simulink model "Lab6_task"  (R2021a)
settings: Solver=VariableStepAuto  StartTime=0.0  StopTime=10.0  RelTol=1e-3
libraries: dspsrcs4 x3
settings Model: Creator=Syed Mujahid Abbas  LastModifiedBy=hp
settings SolverCC: AlgebraicLoopSolver=TrustRegion
settings DataIOCC: ReturnWorkspaceOutputs=off
settings DebuggingCC: SFMachineParentedDataDiag=warning  ArithmeticOperatorsInVariantConditions=warning
settings SFSimCC: SimUseLocalCustomCode=off  CustomCodeUndefinedFunction=UseInterfaceOnly
settings RTWCC: RTWUseLocalCustomCode=off

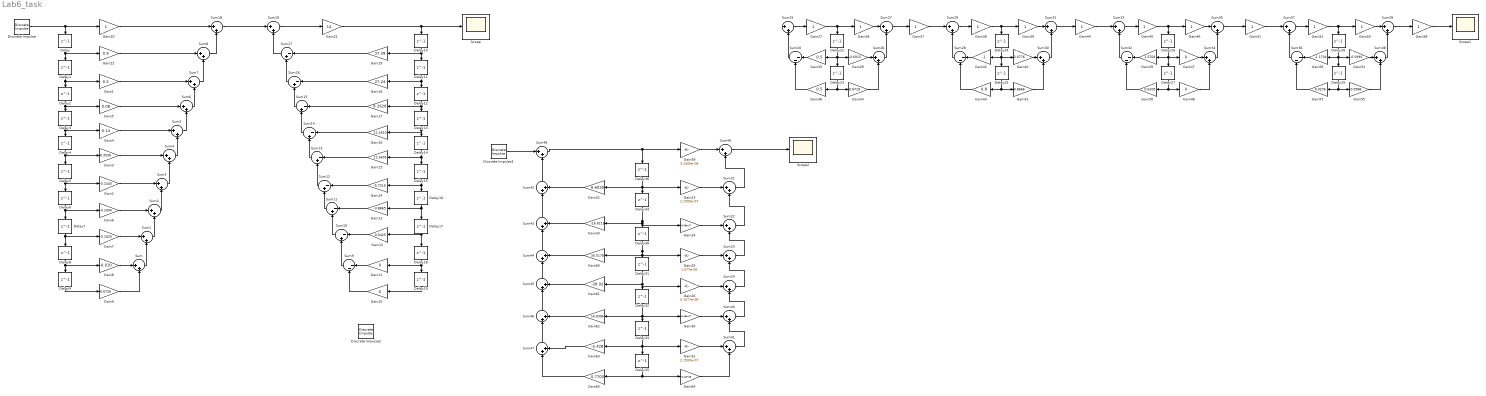
== system Lab6_task ==
  Delay{,1..19,22..36} (35 alike) : Delay  DelayLength=1  InitialCondition=0
  Discrete Impulse : dspsrcs4/Discrete  Impulse  Delay=0  SampleTime=1  FrameSample=1  OutputFrames=off  dataType=double  isSigned=on  wordLen=16  udDataType=sfix(16)  fracBitsMode=Best precision  numFracBits=15  OutDataTypeStr=double  LastOutDataTypeStr=double
  Discrete Impulse2 : dspsrcs4/Discrete  Impulse  Delay=0  SampleTime=1  FrameSample=1  OutputFrames=off  dataType=double  isSigned=on  wordLen=16  udDataType=sfix(16)  fracBitsMode=Best precision  numFracBits=15  OutDataTypeStr=double  LastOutDataTypeStr=double
  Discrete Impulse3 : dspsrcs4/Discrete  Impulse  Delay=0  SampleTime=1  FrameSample=1  OutputFrames=off  dataType=double  isSigned=on  wordLen=16  udDataType=sfix(16)  fracBitsMode=Best precision  numFracBits=15  OutDataTypeStr=double  LastOutDataTypeStr=double
  Gain1 : Gain  Gain=0.5
  Gain{10..11,47..48} (4 alike) : Gain  Gain=0
  Gain12 : Gain  Gain=0.5425
  Gain13 : Gain  Gain=-3.8865
  Gain14 : Gain  Gain=-5.7215
  Gain15 : Gain  Gain=11.6605
  Gain16 : Gain  Gain=12.4810
  Gain17 : Gain  Gain=6.2620
  Gain18 : Gain  Gain=27.24
  Gain19 : Gain  Gain=37.39
  Gain2 : Gain  Gain=-0.2440
  Gain{20,27..28,37..39,44..46,51..53,58} (13 alike) : Gain
  Gain21 : Gain  Gain=14
  Gain22 : Gain  Gain=0.9
  Gain23 : Gain  Gain=2.1500e-07
  Gain24 : Gain  Gain=6.46e-07
  Gain25 : Gain  Gain=1.077e-06
  Gain26 : Gain  Gain=0.1077e-06
  Gain29 : Gain  Gain=-0.6915
  Gain3 : Gain  Gain=0.3530
  Gain30 : Gain  Gain=6.46e-07
  Gain31 : Gain  Gain=2.1500e-07
  Gain32 : Gain  Gain=6.6030
  Gain33 : Gain  Gain=-18.8215
  Gain34 : Gain  Gain=0.6719
  Gain35 : Gain  Gain=0.5
  Gain36 : Gain  Gain=0.5
  Gain4 : Gain  Gain=0.14
  Gain40 : Gain  Gain=2.0776
  Gain41 : Gain  Gain=0.8666
  Gain42 : Gain  Gain=-1
  Gain43 : Gain  Gain=0.8
  Gain49 : Gain  Gain=1.5704
  Gain5 : Gain  Gain=0.08
  Gain50 : Gain  Gain=0.6105
  Gain54 : Gain  Gain=-0.5990
  Gain55 : Gain  Gain=0.0588
  Gain56 : Gain  Gain=-1.1704
  Gain57 : Gain  Gain=0.3276
  Gain59 : Gain  Gain=3.1000e-08
  Gain6 : Gain  Gain=-0.2890
  Gain60 : Gain  Gain=30.0178
  Gain61 : Gain  Gain=-28.92
  Gain62 : Gain  Gain=16.8386
  Gain63 : Gain  Gain=-5.428
  Gain64 : Gain  Gain=3.11e-08
  Gain65 : Gain  Gain=0.7703
  Gain7 : Gain  Gain=-0.1820
  Gain8 : Gain  Gain=-0.010
  Gain9 : Gain  Gain=0.0720
  Scope : Scope
  Scope1 : Scope
  Scope2 : Scope
  Sum{,1..8,18..19,21..27,29..31,33..35,37..49} (37 alike) : Sum  Inputs=|++
  Sum{10..17} (8 alike) : Sum  Inputs=|-+
  Sum{9,20,28,32,36} (5 alike) : Sum  Inputs=|--
  wires:
  Delay6/1 -> Delay7/1, Gain6/1
  Delay5/1 -> Gain2/1, Delay6/1
  Delay9/1 -> Gain9/1
  Delay8/1 -> Gain8/1, Delay9/1
  Delay7/1 -> Gain7/1, Delay8/1
  Sum/1 -> Sum1/2
  Gain6/1 -> Sum2/1
  Sum1/1 -> Sum2/2
  Delay4/1 -> Gain3/1, Delay5/1
  Delay3/1 -> Gain4/1, Delay4/1
  Delay2/1 -> Gain5/1, Delay3/1
  Delay1/1 -> Gain1/1, Delay2/1
  Delay/1 -> Gain22/1, Delay1/1
  Sum2/1 -> Sum3/2
  Gain2/1 -> Sum3/1
  Sum3/1 -> Sum4/2
  Sum4/1 -> Sum5/2
  Sum5/1 -> Sum6/2
  Sum6/1 -> Sum7/2
  Sum7/1 -> Sum8/2
  Delay18/1 -> Gain11/1, Delay19/1
  Delay19/1 -> Gain10/1
  Delay17/1 -> Gain12/1, Delay18/1
  Delay16/1 -> Gain13/1, Delay17/1
  Delay15/1 -> Gain14/1, Delay16/1
  Delay14/1 -> Gain15/1, Delay15/1
  Delay13/1 -> Gain16/1, Delay14/1
  Delay12/1 -> Gain17/1, Delay13/1
  Delay11/1 -> Gain18/1, Delay12/1
  Delay10/1 -> Gain19/1, Delay11/1
  Sum9/1 -> Sum10/2
  Sum10/1 -> Sum11/2
  Sum11/1 -> Sum12/2
  Sum12/1 -> Sum13/2
  Sum13/1 -> Sum14/2
  Sum14/1 -> Sum15/2
  Sum15/1 -> Sum16/2
  Sum16/1 -> Sum17/2
  Sum8/1 -> Sum18/2
  Sum17/1 -> Sum19/2
  Sum18/1 -> Sum19/1
  Discrete Impulse/1 -> Delay/1, Gain20/1
  Sum19/1 -> Gain21/1
  Gain3/1 -> Sum4/1
  Gain4/1 -> Sum5/1
  Gain5/1 -> Sum6/1
  Gain1/1 -> Sum7/1
  Gain22/1 -> Sum8/1
  Gain20/1 -> Sum18/1
  Gain7/1 -> Sum1/1
  Gain8/1 -> Sum/1
  Gain9/1 -> Sum/2
  Gain21/1 -> Delay10/1, Scope/1
  Gain10/1 -> Sum9/2
  Gain11/1 -> Sum9/1
  Gain12/1 -> Sum10/1
  Gain13/1 -> Sum11/1
  Gain14/1 -> Sum12/1
  Gain15/1 -> Sum13/1
  Gain16/1 -> Sum14/1
  Gain17/1 -> Sum15/1
  Gain18/1 -> Sum16/1
  Gain19/1 -> Sum17/1
  Sum26/1 -> Sum27/2
  Gain28/1 -> Sum27/1
  Gain34/1 -> Sum26/2
  Gain29/1 -> Sum26/1
  Sum25/1 -> Gain27/1
  Sum20/1 -> Sum25/2
  Gain35/1 -> Sum20/1
  Gain36/1 -> Sum20/2
  Delay23/1 -> Gain34/1, Gain36/1
  Delay22/1 -> Delay23/1, Gain29/1, Gain35/1
  Gain27/1 -> Gain28/1, Delay22/1
  Gain38/1 -> Delay24/1, Gain39/1
  Delay24/1 -> Gain42/1, Gain40/1, Delay25/1
  Delay25/1 -> Gain43/1, Gain41/1
  Gain43/1 -> Sum28/2
  Gain42/1 -> Sum28/1
  Gain37/1 -> Sum29/1
  Sum28/1 -> Sum29/2
  Sum29/1 -> Gain38/1
  Gain40/1 -> Sum30/1
  Gain41/1 -> Sum30/2
  Gain39/1 -> Sum31/1
  Sum30/1 -> Sum31/2
  Sum27/1 -> Gain37/1
  Sum34/1 -> Sum35/2
  Gain46/1 -> Sum35/1
  Gain48/1 -> Sum34/2
  Gain47/1 -> Sum34/1
  Sum33/1 -> Gain45/1
  Sum32/1 -> Sum33/2
  Gain44/1 -> Sum33/1
  Gain49/1 -> Sum32/1
  Gain50/1 -> Sum32/2
  Delay27/1 -> Gain48/1, Gain50/1
  Delay26/1 -> Delay27/1, Gain47/1, Gain49/1
  Gain45/1 -> Gain46/1, Delay26/1
  Sum31/1 -> Gain44/1
  Sum35/1 -> Gain51/1
  Gain52/1 -> Delay28/1, Gain53/1
  Delay28/1 -> Gain56/1, Gain54/1, Delay29/1
  Delay29/1 -> Gain57/1, Gain55/1
  Gain57/1 -> Sum36/2
  Gain56/1 -> Sum36/1
  Gain51/1 -> Sum37/1
  Sum36/1 -> Sum37/2
  Sum37/1 -> Gain52/1
  Gain54/1 -> Sum38/1
  Gain55/1 -> Sum38/2
  Gain53/1 -> Sum39/1
  Sum38/1 -> Sum39/2
  Sum39/1 -> Gain58/1
  Gain58/1 -> Scope1/1
  Delay36/1 -> Gain23/1, Gain32/1, Delay34/1
  Delay34/1 -> Gain33/1, Gain24/1, Delay30/1
  Delay30/1 -> Gain60/1, Gain25/1, Delay31/1
  Delay31/1 -> Gain61/1, Gain26/1, Delay32/1
  Delay32/1 -> Gain62/1, Gain30/1, Delay33/1
  Delay33/1 -> Delay35/1, Gain63/1, Gain31/1
  Delay35/1 -> Gain65/1, Gain64/1
  Gain23/1 -> Sum21/1
  Gain65/1 -> Sum47/1
  Gain63/1 -> Sum47/2
  Sum47/1 -> Sum46/1
  Gain62/1 -> Sum46/2
  Sum46/1 -> Sum45/1
  Gain61/1 -> Sum45/2
  Sum45/1 -> Sum44/1
  Gain60/1 -> Sum44/2
  Sum44/1 -> Sum43/1
  Gain33/1 -> Sum43/2
  Sum43/1 -> Sum42/1
  Gain32/1 -> Sum42/2
  Sum22/1 -> Sum21/2
  Gain24/1 -> Sum22/1
  Gain25/1 -> Sum23/1
  Gain26/1 -> Sum24/1
  Gain30/1 -> Sum40/1
  Gain31/1 -> Sum41/1
  Gain64/1 -> Sum41/2
  Sum41/1 -> Sum40/2
  Sum40/1 -> Sum24/2
  Sum24/1 -> Sum23/2
  Sum23/1 -> Sum22/2
  Sum42/1 -> Sum48/2
  Discrete Impulse3/1 -> Sum48/1
  Sum48/1 -> Gain59/1, Delay36/1
  Gain59/1 -> Sum49/1
  Sum21/1 -> Sum49/2
  Sum49/1 -> Scope2/1
